simulink model "Reconstructing"  (R2016a)
settings: Solver=VariableStepAuto  StartTime=0.0  StopTime=0  RelTol=1e-3
values from neighbouring files (symbols this model uses):
  data = zeros(row,mem + 2 + 1)    [Cepstrum_Compression.m]    (also in Cepstrum_Compression_Simulink.m = data.Data)
  mem = col - 3    [Cepstrum_Compression.m]    (also in Cepstrum_Compression_Simulink.m)
  N = data(1,end)    [Cepstrum_Compression.m]    (also in Cepstrum_Compression_Simulink.m)
libraries: dspsigops x2, dspmtrx3 x2
settings Model: Creator=HP  LastModifiedBy=HP

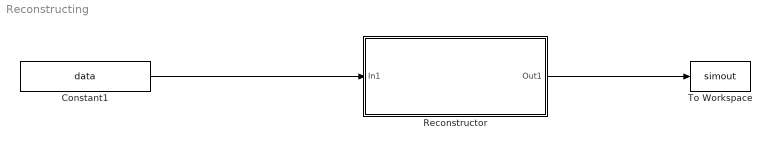
== system Reconstructing ==
  Constant1 : Constant  Value=data
  Reconstructor : Subsystem
  To Workspace : ToWorkspace  VariableName=simout  SaveFormat=Structure  SampleTime=-1
  wires:
  Constant1/1 -> Reconstructor/1(In1)
  Reconstructor/1(Out1) -> To Workspace/1

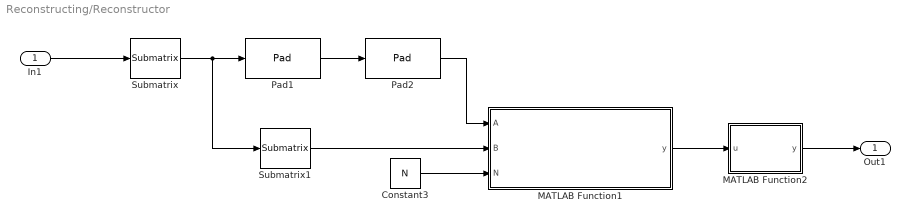
== system Reconstructing/Reconstructor ==
  In1 : Inport
  Constant3 : Constant  Value=N
  MATLAB Function1 : MATLAB Function  TreatAsAtomicUnit=on
  MATLAB Function2 : MATLAB Function  TreatAsAtomicUnit=on
  Pad1 : dspsigops/Pad  padAlong=Rows  dimsToPad=1  valSrc=Specify via dialog  padVal=0  spec=Output size  padNumOutRowsSpecMethod=User-specified  numOutRows=row  padNumOutColsSpecMethod=User-specified  numOutCols=mem  isVarDimsMode=off  padBeginning=0  padEnd=0  outSizeMode=User-specified  outSize=1  padSigAt=End  trunc_flag=None  roundingMode=Floor  overflowMode=off  truncOrWrapMode=Truncate  wrap_flag=None
  Pad2 : dspsigops/Pad  padAlong=Rows  dimsToPad=1  valSrc=Specify via dialog  padVal=0  spec=Output size  padNumOutRowsSpecMethod=User-specified  numOutRows=row  padNumOutColsSpecMethod=User-specified  numOutCols=N  isVarDimsMode=off  padBeginning=0  padEnd=0  outSizeMode=User-specified  outSize=1  padSigAt=End  trunc_flag=None  roundingMode=Floor  overflowMode=off  truncOrWrapMode=Truncate  wrap_flag=None
  Submatrix : dspmtrx3/Submatrix  RowSpan=Range of rows  RowStartMode=Index  RowStartIndex=i  RowEndMode=Index  RowEndIndex=i  ColSpan=Range of columns  ColStartMode=First  ColStartIndex=1  ColEndMode=Last  ColEndIndex=1
  Submatrix1 : dspmtrx3/Submatrix  RowSpan=Range of rows  RowStartMode=First  RowStartIndex=1  RowEndMode=Last  RowEndIndex=1  ColSpan=Range of columns  ColStartMode=Index  ColStartIndex=mem+1  ColEndMode=Last  ColEndIndex=1
  Out1 : Outport
  wires:
  MATLAB Function1/1(y) -> MATLAB Function2/1(u)
  Submatrix1/1 -> MATLAB Function1/2(B)
  Constant3/1 -> MATLAB Function1/3(N)
  Submatrix/1 -> Submatrix1/1, Pad1/1
  In1/1 -> Submatrix/1
  Pad2/1 -> MATLAB Function1/1(A)
  Pad1/1 -> Pad2/1
  MATLAB Function2/1(y) -> Out1/1

== matlab function Reconstructing/Reconstructor/MATLAB Function1 ==
  data: A input; y output; B input; N input
function y = assign_peak(A,B,N)
%#codegen
[m,n] = size(A);
y = zeros(m,n);
loc = B(2);
val = B(1);
A(loc) = val;
A = 2.*A;
A(1) = 0.5.*A(1);
A(N/2) = 0.5.*A(N/2);
y = A;

== matlab function Reconstructing/Reconstructor/MATLAB Function2 ==
  data: u input; y output
function y = inv_cepstrum(u)
coder.extrinsic('icceps')
y = zeros(length(u),1);
y = icceps(u,0);
